simulink model "bili"  (R2023a)
settings: Solver=VariableStepAuto  StartTime=0.0  StopTime=1000000  RelTol=1e-3
settings Model: Creator=17634948724  LastModifiedBy=17634948724

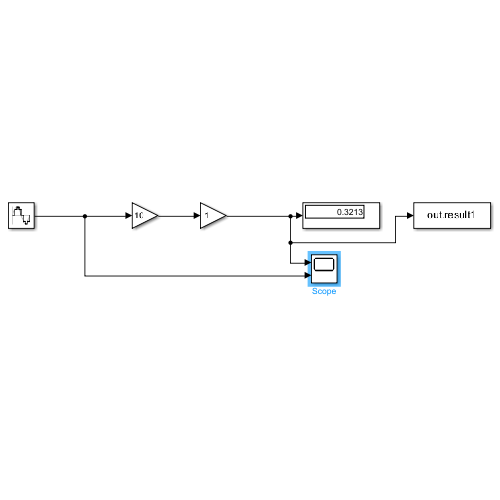
[thumbnail: Simulink's stored preview of the top-level diagram]
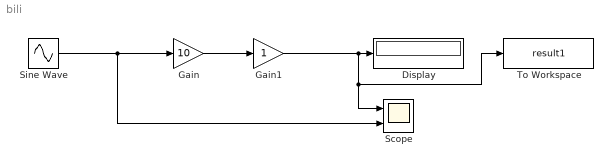
== system bili ==
  Display : Display
  Gain : Gain  Gain=10
  Gain1 : Gain
  Scope : Scope  NumInputPorts=2
  Sine Wave : Sin  Amplitude=0.05  Frequency=628.3185  SampleTime=0.1
  To Workspace : ToWorkspace  VariableName=result1  SaveFormat=Timeseries  SampleTime=-1
  wires:
  Gain/1 -> Gain1/1
  Gain1/1 -> To Workspace/1, Scope/1, Display/1
  Sine Wave/1 -> Scope/2, Gain/1
